simulink model "ofdm_13"  (Simulink 7.4)
settings: Solver=FixedStepDiscrete  SolverMode=SingleTasking  StartTime=0.0  StopTime=inf  MaxStep=1/(100*40e6)  RelTol=1e-3
PreLoadFcn:
  | Fsymbol              = .5e6;         % Symbol rate
  | D=8;  % decimation / interpolation
  | Bits_per_Symbol = 2;
  | Fbit  = Bits_per_Symbol*Fsymbol;
  | 
  | FFT_Size  = 64;
  | Cyclic        = 16;
  | Pilots         = 16;
  | Pilot_Level = 8;
  | Zero_Pad  = 3;
  | QAM_Level = 6;
  | 
  | OFDM_Frame =  FFT_Size+Cyclic;
  | Symbols_per_Frame = FFT_Size-Pilots-Zero_Pad;
  | 
  | Bits_per_Frame = Bits_per_Symbol*Symbols_per_Frame;
  | 
  | F_nco = Fsymbol*D*OFDM_Frame/(Symbols_per_Frame);
  | nco_nominal=2/D;
  | 
  | 
  | Fdelay = 8;  % rrc filter delay
  | Alpha = .25;  % excess BW
  | rrc_coef=rcosine(1,D,'fir/sqrt',Alpha,Fdelay);
  | rrc_coef=rrc_coef/sum(rrc_coef);
  | 
  | 
  | % coefficents for Farrow filter
  | b3 = [1/6 -1/2  1/2 -1/6];
  | b2 = [1/2 -1    1/2  0];
  | b1 = [1/3  1/2 -1    1/6];
  | b0 = [0    1    0    0];
StartFcn:
  | tic
StopFcn:
  | trun=toc
values from neighbouring files (symbols this model uses):
  Fs = 1    [16 qam.m]    (also in G.m = input('Enter sampling frequency='))
  j = imread('lena.jpg')    [ansk3.m]    (also in cosine_filter.m = 2; imag1.m)
  N = [N1;N2;N1_;N2_]    [FFT_OFDM_MIMO.m]    (also in MRCplot.m = 1000000; SDplot.m = 1000000; ansk2.m = 10; ansk3.m = 10)
undefined symbols (not defined in the file or in its folder): dBW, dfilt, Hz, magnitude, sided, Ts, Two
libraries: simulink x25, dspobslib x22, dspsigops x13, dspbuff3 x5, dspsnks4 x4, dspxfrm3 x4, dspstat3 x4, commsink2 x3, commchan3 x2, dsparch4 x2, commrandsrc2 x2, commdigbbndam3 x2
(part 1 of 2)
Description:
  | Pilot Driven OFDM  Synchronization
settings Model: Creator=Dick Benson  LastModifiedBy=Dick
settings Model: ModifiedHistory=|
  | 12/8/07  D&C
  | 12/03/08  Added BER, tuned control loops, enhanced channel model.
settings DataIOCC: SaveOutput=off  SignalLogging=off  SaveTime=off  SignalLoggingName=sigsOut
settings OptimizationCC: BlockReduction=off  BooleanDataType=off  InlineInvariantSignals=on  InitFltsAndDblsToZero=on
settings DebuggingCC: SaveWithParameterizedLinksMsg=none  SignalResolutionControl=TryResolveAllWithWarning  SolverPrmCheckMsg=none  InheritedTsInSrcMsg=none  MultiTaskDSMMsg=warning  MultiTaskCondExecSysMsg=none  ParameterPrecisionLossMsg=none  StrictBusMsg=None
settings HardwareCC: TargetUnknown=on
settings RTWCC: IncludeERTFirstTime=on
settings GRTTargetCC: TargetFcnLib=ansi_tfl_tmw.mat

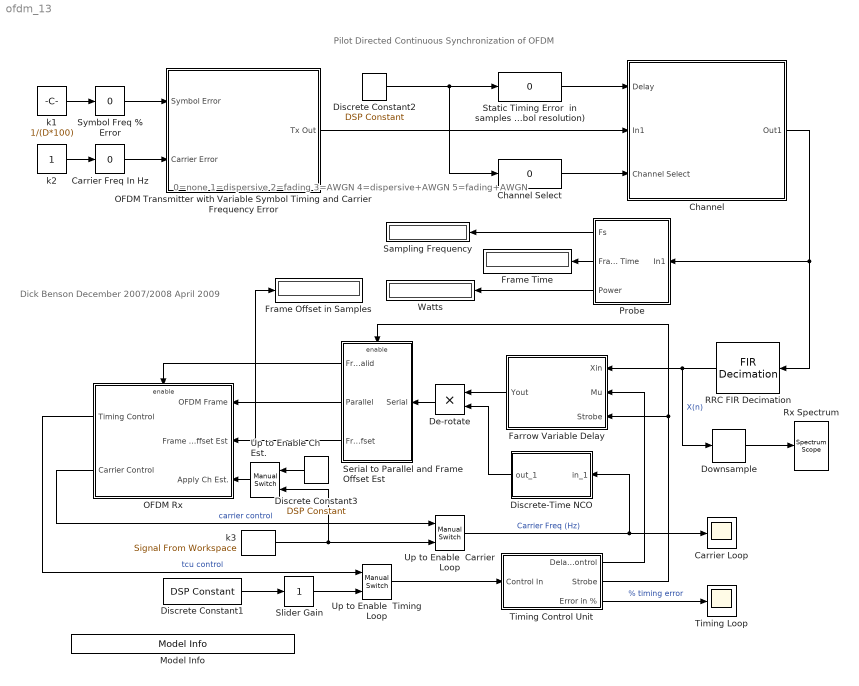
== system ofdm_13 ==
  note: Pilot Directed Continuous Synchronization of OFDM
  note: Dick Benson
      | December 2007/2008
      | April 2009
  note: 0=none
      | 1=dispersive
      | 2=fading
      | 3=AWGN
      | 4=dispersive+AWGN
      | 5=fading+AWGN
  Carrier Freq In Hz : simulink/Math Operations/Slider Gain  SystemSampleTime=-1  low=-1000  gain=0  high=1000
  Carrier Loop : Scope
      settings: TimeRange=0.008999999999999999  YMin=-1000  YMax=1000  MaxDataPoints=50000  Decimation=4
  Channel : Subsystem
  Channel Select : simulink/Math Operations/Slider Gain  SystemSampleTime=-1  low=0  gain=0  high=5
  De-rotate : Product  OutDataType=sfix(16)  OutScaling=2^0  RndMeth=Zero
  Discrete Constant1 : dspobslib/DSP Constant  SystemSampleTime=-1  Value=nco_nominal  SampleMode=Discrete  discreteOutput=Sample-based (interpret vectors as 1-D)  continuousOutput=Sample-based  sampTime=2/F_nco  framePeriod=2/F_nco  dataType=Inherit via back propagation  isSigned=on  wordLen=16  udDataType=sfix(16)  fracBitsMode=Best precision  numFracBits=15  InterpretAs1D=on  Ts=2/F_nco  FramebasedOutput=off
      settings: additionalParams=on
  Discrete Constant2 : dspobslib/DSP Constant  SystemSampleTime=-1  Value=1  SampleMode=Discrete  discreteOutput=Sample-based (interpret vectors as 1-D)  continuousOutput=Sample-based  sampTime=inf  framePeriod=inf  dataType=Inherit via back propagation  isSigned=on  wordLen=16  udDataType=sfix(16)  fracBitsMode=Best precision  numFracBits=15  InterpretAs1D=on  Ts=inf  FramebasedOutput=off
      settings: additionalParams=on
  Discrete Constant3 : dspobslib/DSP Constant  SystemSampleTime=-1  Value=1  SampleMode=Discrete  discreteOutput=Sample-based (interpret vectors as 1-D)  continuousOutput=Sample-based  sampTime=inf  framePeriod=inf  dataType=Inherit via back propagation  isSigned=on  wordLen=16  udDataType=sfix(16)  fracBitsMode=Best precision  numFracBits=15  InterpretAs1D=on  Ts=inf  FramebasedOutput=off
      settings: additionalParams=on
  Discrete-Time NCO : Subsystem  mask(Discrete-Time VCO){Ac=1, Fc=0, Kc=1, Ph=0, ts=2/F_nco}
      mask prompts: Ac "Output amplitude:"; Fc "Oscillation frequency (Hz):"; Kc "Input sensitivity:"; Ph "Initial phase (rad):"; ts "Sample time:"
      mask help: Generate a discrete-time output signal whose frequency changes in response to the amplitude variations of the input signal. The input signal must be a scalar.
      mask init:
      | if ((length(Ac)~=1) | (length(Fc)~=1) | (length(Kc)~=1) | (length(Ph)~=1) | (length(ts)~=1) |(length(Ph)~=1))error('Mask parameters must be scalar values.');end;
      | pi2=2*pi;
      mask Help: helpview(commbhelp)
      mask Display: disp('Discrete-Time\nNCO (rab)')
  Downsample : dspsigops/Downsample  N=D/2  phase=0  ic=0  smode=Allow multirate  fmode=Maintain input frame size
  Farrow Variable Delay : Subsystem
  Frame Offset in Samples : Display
  Frame Time : Display
  Model Info : simulink/Model-Wide Utilities/Model Info  SystemSampleTime=-1  InitialBlockCM=none  BlockCM=none  Frame=on  DisplayStringWithTags=Copywrite 2008-2010 The MathWorks, Inc.  HorizontalTextAlignment=Center  LeftAlignmentValue=0.5  SourceBlockDiagram=ofdm_13  TagMaxNumber=20
  OFDM Rx : Subsystem
  OFDM Transmitter with Variable Symbol Timing and Carrier Frequency Error : Subsystem
  Probe : Subsystem
  RRC FIR Decimation : dspmlti4/FIR Decimation  DialogController=dspdialog.FIRDecimation  DialogControllerArgs=DataTag16  h=rrc_coef  D=D/4  filtStruct=Direct form  framing=Maintain input frame rate  outputBufInitCond=0  roundingMode=Floor  overflowMode=off  FilterSource=Specify via dialog  FilterObject=Hm_firdecim
  Rx Spectrum : dspsnks4/Spectrum Scope  DialogController=dspdialog.SpectrumScope  DialogControllerArgs=DataTag17  SystemSampleTime=-1  ScopeProperties=on  Domain=Frequency  HorizSpan=1  UseBuffer=on  BufferSize=80  Overlap=0  inpFftLenInherit=on  FFTlength=256  numAvg=10  DisplayProperties=off  AxisGrid=on  Memory=off  FrameNumber=on  AxisLegend=off  AxisZoom=off  OpenScopeAtSimStart=on  OpenScopeImmediately=off  FigPos=[623 549 194 174]  AxisProperties=off  XUnits=Hertz  XRange=Two-sided ((-Fs/2...Fs/2])  XDisplay=0  InheritXIncr=on  XIncr=1.0  XLabel=Samples  XLimit=Auto  YUnits=dBW/Hertz  XMax=1  XMin=0  YLabel=dBW/Hz  LineProperties=off  wintypeSpecScope=Boxcar  RsSpecScope=50  betaSpecScope=5  winsampSpecScope=Periodic  XAxisParamsVer=6.8
      settings: YMin=-79.4885  YMax=-44.4885
  Sampling Frequency : Display
  Serial to Parallel and Frame Offset Est : Subsystem  TreatAsAtomicUnit=on
  Slider Gain : simulink/Math Operations/Slider Gain  SystemSampleTime=-1  low=0.99  gain=1  high=1.01
  Static Timing Error  in samples (1/8 symbol resolution) : simulink/Math Operations/Slider Gain  SystemSampleTime=-1  low=-40  gain=0  high=40
  "Symbol Freq % Error " : simulink/Math Operations/Slider Gain  SystemSampleTime=-1  low=-0.5  gain=0  high=0.5
  Timing Control Unit : Subsystem
  Timing Loop : Scope
      settings: TimeRange=0.008999999999999999  YMin=-0.5  YMax=0.5  MaxDataPoints=50000
  Up to Enable  Carrier Loop : simulink/Signal Routing/Manual Switch  SystemSampleTime=-1  sw=0  action=0  varsize=off
  Up to Enable Ch Est. : simulink/Signal Routing/Manual Switch  SystemSampleTime=-1  sw=0  action=0  varsize=off
  Up to Enable  Timing Loop : simulink/Signal Routing/Manual Switch  SystemSampleTime=-1  sw=0  action=0  varsize=off
  Watts : Display
  k1 : Constant  Value=1/(D*100)  OutDataType=sfix(16)  OutScaling=2^0
  k2 : Constant  OutDataType=sfix(16)  OutScaling=2^0
  k3 : dspsrcs4/Signal From Workspace  SystemSampleTime=-1  X=0  Ts=-1  nsamps=1  OutputAfterFinalValue=Holding final value  ignoreOrWarnInputAndFrameLengths=off
  wires:
  k1/1 -> "Symbol Freq % Error "/1
  "Symbol Freq % Error "/1 -> OFDM Transmitter with Variable Symbol Timing and Carrier Frequency Error/1(Symbol Error)
  Carrier Freq In Hz/1 -> OFDM Transmitter with Variable Symbol Timing and Carrier Frequency Error/2(Carrier Error)
  k2/1 -> Carrier Freq In Hz/1
  Probe/1(Fs) -> Sampling Frequency/1
  OFDM Transmitter with Variable Symbol Timing and Carrier Frequency Error/1(Tx Out) -> Channel/2(In1)
  Timing Control Unit/1(Delay Control) -> Farrow Variable Delay/2(Mu)
  Timing Control Unit/2(Strobe) -> Farrow Variable Delay/3(Strobe), Serial to Parallel and Frame Offset Est/Enable
  Discrete Constant1/1 -> Slider Gain/1
  RRC FIR Decimation/1 -> Farrow Variable Delay/1(Xin), Downsample/1  "X(n)"
  Channel/1(Out1) -> RRC FIR Decimation/1, Probe/1(In1)
  Probe/3(Power) -> Watts/1
  Probe/2(Frame Time) -> Frame Time/1
  Discrete Constant2/1 -> Static Timing Error  in samples (1/8 symbol resolution)/1, Channel Select/1
  Static Timing Error  in samples (1/8 symbol resolution)/1 -> Channel/1(Delay)
  OFDM Rx/1(Timing Control) -> Up to Enable  Timing Loop/1  "tcu control"
  Up to Enable  Timing Loop/1 -> Timing Control Unit/1(Control In)
  Discrete-Time NCO/1(out_1) -> De-rotate/2
  De-rotate/1 -> Serial to Parallel and Frame Offset Est/1(Serial)
  Farrow Variable Delay/1(Yout) -> De-rotate/1
  Timing Control Unit/3(Error in %) -> Timing Loop/1  "% timing error"
  Downsample/1 -> Rx Spectrum/1
  Serial to Parallel and Frame Offset Est/2(Parallel) -> OFDM Rx/1(OFDM Frame)
  Serial to Parallel and Frame Offset Est/3(Frame Offset) -> OFDM Rx/2(Frame Offset Est), Frame Offset in Samples/1
  Slider Gain/1 -> Up to Enable  Timing Loop/2
  OFDM Rx/2(Carrier Control) -> Up to Enable  Carrier Loop/1  "carrier control"
  Up to Enable  Carrier Loop/1 -> Discrete-Time NCO/1(in_1), Carrier Loop/1  "Carrier Freq (Hz)"
  k3/1 -> Up to Enable  Carrier Loop/2, Up to Enable Ch Est./2
  Serial to Parallel and Frame Offset Est/1(FrameValid) -> OFDM Rx/Enable
  Up to Enable Ch Est./1 -> OFDM Rx/3(Apply Ch Est.)
  Discrete Constant3/1 -> Up to Enable Ch Est./1
  Channel Select/1 -> Channel/3(Channel Select)

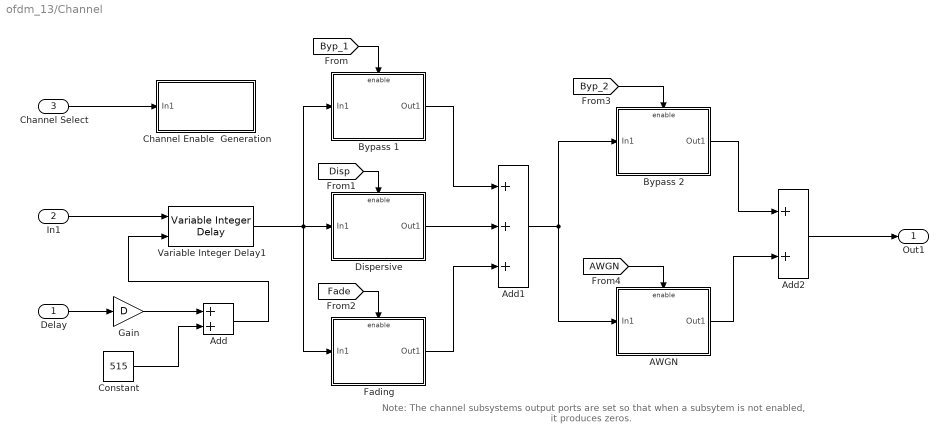
== system ofdm_13/Channel ==
  note: Note: The channel subsystems output ports are set so that
      | when a subsytem is not enabled, it produces zeros.
  Delay : Inport  OutDataType=sfix(16)  OutScaling=2^0
  In1 : Inport  Port=2  OutDataType=sfix(16)  OutScaling=2^0
  Channel Select : Inport  Port=3  OutDataType=sfix(16)  OutScaling=2^0
  AWGN : Subsystem  TreatAsAtomicUnit=on
  Add : Sum  OutDataType=sfix(16)  OutScaling=2^-10
  Add1 : Sum  Inputs=+++  OutDataType=sfix(16)  OutScaling=2^-10
  Add2 : Sum  OutDataType=sfix(16)  OutScaling=2^-10
  Bypass 1 : Subsystem  TreatAsAtomicUnit=on
  Bypass 2 : Subsystem  TreatAsAtomicUnit=on
  Channel Enable  Generation : Subsystem
  Constant : Constant  Value=515  OutDataType=sfix(16)  OutScaling=2^0
  Dispersive : Subsystem  TreatAsAtomicUnit=on
  Fading : Subsystem  TreatAsAtomicUnit=on
  Gain : Gain  Gain=D  ParameterDataType=sfix(16)  ParameterScaling=2^0  OutDataType=sfix(16)  OutScaling=2^0
  Variable Integer Delay1 : dspsigops/Variable Integer Delay  dmax=2*516  ic=0  noDFT=off
  Out1 : Outport  OutDataType=sfix(16)  OutScaling=2^0
  wires:
  Delay/1 -> Gain/1
  Constant/1 -> Add/2
  Gain/1 -> Add/1
  Dispersive/1(Out1) -> Add1/2
  Bypass 1/1(Out1) -> Add1/1
  Fading/1(Out1) -> Add1/3
  Add1/1 -> AWGN/1(In1), Bypass 2/1(In1)
  Bypass 2/1(Out1) -> Add2/1
  AWGN/1(Out1) -> Add2/2
  Add2/1 -> Out1/1
  Channel Select/1 -> Channel Enable  Generation/1(In1)
  [Byp_1] -> Bypass 1/Enable
  [Disp] -> Dispersive/Enable
  [Fade] -> Fading/Enable
  [Byp_2] -> Bypass 2/Enable
  [AWGN] -> AWGN/Enable
  Variable Integer Delay1/1 -> Dispersive/1(In1), Bypass 1/1(In1), Fading/1(In1)
  In1/1 -> Variable Integer Delay1/1
  Add/1 -> Variable Integer Delay1/2

== system ofdm_13/Discrete-Time NCO ==
  note: Amplitude
  note: Phase Accumulator
      | Modulus
  note: Center Freq
  note: VCO Sensitivity
  note: initial condx=Ph
  in_1 : Inport  OutDataType=sfix(16)  OutScaling=2^0
  Discrete Constant1 : dspobslib/DSP Constant  SystemSampleTime=-1  Value=Fc*pi2*ts  SampleMode=Discrete  discreteOutput=Sample-based (interpret vectors as 1-D)  continuousOutput=Sample-based  sampTime=ts  framePeriod=ts  dataType=Inherit via back propagation  isSigned=on  wordLen=16  udDataType=sfix(16)  fracBitsMode=Best precision  numFracBits=15  InterpretAs1D=on  Ts=ts  FramebasedOutput=off
      settings: additionalParams=on
  Discrete Constant2 : dspobslib/DSP Constant  SystemSampleTime=-1  Value=pi2  SampleMode=Discrete  discreteOutput=Sample-based (interpret vectors as 1-D)  continuousOutput=Sample-based  sampTime=ts  framePeriod=ts  dataType=Inherit via back propagation  isSigned=on  wordLen=16  udDataType=sfix(16)  fracBitsMode=Best precision  numFracBits=15  InterpretAs1D=on  Ts=ts  FramebasedOutput=off
      settings: additionalParams=on
  Math Function : Math  Operator=mod  OutDataType=sfix(16)  OutScaling=2^0  SaturateOnIntegerOverflow=on
  Real-Imag to Complex : RealImagToComplex
  Sensitivity : Gain  Gain=Kc*pi2*ts  ParameterDataType=sfix(16)  ParameterScaling=2^0  OutDataType=sfix(16)  OutScaling=2^0  SaturateOnIntegerOverflow=on  OutDataTypeStr=Inherit: Same as input  ParamDataTypeStr=Inherit: Same as input
  Sensitivity2 : Gain  Gain=Ac  ParameterDataType=sfix(16)  ParameterScaling=2^0  OutDataType=sfix(16)  OutScaling=2^0  SaturateOnIntegerOverflow=on  OutDataTypeStr=Inherit: Same as input  ParamDataTypeStr=Inherit: Same as input
  Sum1 : Sum  Inputs=+++  OutDataType=sfix(16)  OutScaling=2^0  SaturateOnIntegerOverflow=on  InputSameDT=on  OutDataTypeStr=Inherit: Same as first input
  Trigonometric Function : Trigonometry  Operator=cos
  Trigonometric Function1 : Trigonometry
  Unit Delay : UnitDelay  X0=Ph  SampleTime=ts
  out_1 : Outport  OutDataType=sfix(16)  OutScaling=2^0  InitialOutput=0
  wires:
  Discrete Constant1/1 -> Sum1/2
  Sensitivity2/1 -> out_1/1
  Trigonometric Function/1 -> Real-Imag to Complex/1
  Unit Delay/1 -> Sum1/3, Trigonometric Function1/1, Trigonometric Function/1
  Sensitivity/1 -> Sum1/1
  in_1/1 -> Sensitivity/1
  Math Function/1 -> Unit Delay/1
  Sum1/1 -> Math Function/1
  Discrete Constant2/1 -> Math Function/2
  Trigonometric Function1/1 -> Real-Imag to Complex/2
  Real-Imag to Complex/1 -> Sensitivity2/1

== system ofdm_13/Farrow Variable Delay ==
  Xin : Inport  OutDataType=sfix(16)  OutScaling=2^0
  Mu : Inport  Port=2  OutDataType=sfix(16)  OutScaling=2^0
  Strobe : Inport  Port=3  OutDataType=sfix(16)  OutScaling=2^0
  Calculate Filter : Subsystem
  Filter State (4x1) : dspbuff3/Buffer  N=4  V=3  ic=0
  Yout : Outport  OutDataType=sfix(16)  OutScaling=2^0
  wires:
  Xin/1 -> Filter State (4x1)/1
  Mu/1 -> Calculate Filter/1(In1)
  Filter State (4x1)/1 -> Calculate Filter/2(In2)
  Calculate Filter/1(Out1) -> Yout/1
  Strobe/1 -> Calculate Filter/Enable

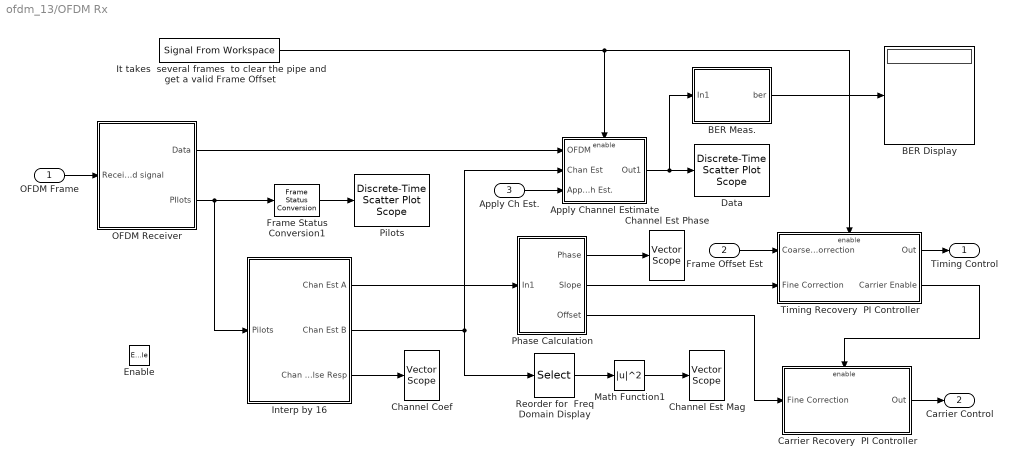
== system ofdm_13/OFDM Rx ==
  OFDM Frame : Inport  OutDataType=sfix(16)  OutScaling=2^0
  Frame Offset Est : Inport  Port=2  OutDataType=sfix(16)  OutScaling=2^0
  Apply Ch Est. : Inport  Port=3  OutDataType=sfix(16)  OutScaling=2^0
  Enable : EnablePort
  Apply Channel Estimate : Subsystem
  BER Display : Display
  BER Meas. : Subsystem
  Carrier Recovery  PI Controller : Subsystem
  Channel Coef : dspsnks4/Vector Scope  DialogController=dspdialog.VectorScope  DialogControllerArgs=DataTag3  ScopeProperties=on  Domain=Time  HorizSpan=1  DisplayProperties=off  AxisGrid=on  Memory=off  FrameNumber=off  AxisLegend=off  AxisZoom=off  OpenScopeAtSimStart=on  OpenScopeImmediately=off  FigPos=[827 549 193 173]  AxisProperties=off  XUnits=Hertz  XRange=[0...Fs/2]  InheritXIncr=on  XIncr=1  XLabel=Time  XLimit=Auto  XMin=0  XMax=1  XStart=0  YUnits=dB  YLabel=Amplitude  LineProperties=off  LineStyles=none|none  LineMarkers=*|*  LineColors=blue | red  XAxisParamsVer=6.8
      settings: YMin=-2  YMax=2
  "Channel Est Mag " : dspsnks4/Vector Scope  DialogController=dspdialog.VectorScope  DialogControllerArgs=DataTag4  ScopeProperties=on  Domain=Frequency  HorizSpan=1  DisplayProperties=off  AxisGrid=on  Memory=off  FrameNumber=on  AxisLegend=off  AxisZoom=off  OpenScopeAtSimStart=on  OpenScopeImmediately=off  FigPos=[624 329 193 172]  AxisProperties=off  XUnits=Hertz  XRange=[-Fs/2...Fs/2]  InheritXIncr=off  XIncr=8/F_nco  XLabel=Time  XLimit=Auto  XMin=0  XMax=1  XStart=0  YUnits=dB  YLabel=Amplitude in dB  LineProperties=off  XAxisParamsVer=6.8
      settings: YMin=-20  YMax=15
  Channel Est Phase : dspsnks4/Vector Scope  DialogController=dspdialog.VectorScope  DialogControllerArgs=DataTag5  ScopeProperties=on  Domain=Frequency  HorizSpan=1  DisplayProperties=off  AxisGrid=on  Memory=off  FrameNumber=off  AxisLegend=off  AxisZoom=off  OpenScopeAtSimStart=on  OpenScopeImmediately=off  FigPos=[827 332 196 169]  AxisProperties=off  XUnits=Hertz  XRange=[-Fs/2...Fs/2]  InheritXIncr=off  XIncr=8/F_nco  XLabel=Time  XLimit=Auto  XMin=0  XMax=1  XStart=0  YUnits=Magnitude  YLabel=Degrees  LineProperties=off  LineColors=blue  XAxisParamsVer=6.8
      settings: YMin=-400  YMax=400
  Data : commsink2/Discrete-Time Scatter Plot Scope  Tag=ScatterPlot  SystemSampleTime=-1  sampPerSymb=1  offsetEye=0  numTraces=100  numNewFrames=10  LineMarkers=square  LineColors=r  fading=off  render=off  AxisGrid=on  xMin=-2  xMax=2  yMin=-2  yMax=2  inphaseLabel=In-phase Amplitude  quadratureLabel=Quadrature Amplitude  openScopeAtSimStart=on  FrameNumber=off  FigPos=[626 82 194 198]  figTitle=Scatter Plot  numLinesMax=8  block_type_=scatter
  Frame Status Conversion1 : dspobslib/Frame Status Conversion  SystemSampleTime=-1  growRefPort=off  outframe=Frame-based
  Interp by 16 : Subsystem
  It takes  several frames  to clear the pipe and get a valid Frame Offset : dspsrcs4/Signal From Workspace  SystemSampleTime=-1  X=[zeros(1,10),1]  Ts=-1  nsamps=1  OutputAfterFinalValue=Holding final value  ignoreOrWarnInputAndFrameLengths=off
  Math Function1 : Math  Operator=magnitude^2  OutDataType=sfix(16)  OutScaling=2^0  SaturateOnIntegerOverflow=on
  OFDM Receiver : Subsystem
      mask Display:
      | disp('OFDM\nReceiver');
      | port_label('output',2,'pilots')
  Phase Calculation : Subsystem
  Pilots : commsink2/Discrete-Time Scatter Plot Scope  Tag=ScatterPlot  SystemSampleTime=-1  sampPerSymb=1  offsetEye=0  numTraces=100  numNewFrames=10  LineMarkers=*  LineColors=r  fading=off  render=off  AxisGrid=on  xMin=-2  xMax=2  yMin=-2  yMax=2  inphaseLabel=In-phase Amplitude  quadratureLabel=Quadrature Amplitude  openScopeAtSimStart=on  FrameNumber=off  FigPos=[828 84 191 197]  figTitle=Scatter Plot  numLinesMax=8  block_type_=scatter
  Reorder for  Freq Domain Display : Selector  InputPortWidth=64  IndexOptions=Index vector (dialog)  Indices=[33:64 1:32]  OutputSizes=1
  Timing Recovery  PI Controller : Subsystem
  Timing Control : Outport  OutDataType=sfix(16)  OutScaling=2^0  InitialOutput=nco_nominal
  Carrier Control : Outport  Port=2  OutDataType=sfix(16)  OutScaling=2^0  InitialOutput=0
  wires:
  OFDM Frame/1 -> OFDM Receiver/1(Received signal)
  OFDM Receiver/2(PIlots) -> Interp by 16/1(Pilots), Frame Status Conversion1/1
  Interp by 16/2(Chan Est B) -> Apply Channel Estimate/2(Chan Est), Reorder for  Freq Domain Display/1
  Reorder for  Freq Domain Display/1 -> Math Function1/1
  Phase Calculation/2(Slope) -> Timing Recovery  PI Controller/2(Fine Correction)
  OFDM Receiver/1(Data) -> Apply Channel Estimate/1(OFDM)
  Phase Calculation/1(Phase) -> Channel Est Phase/1
  Math Function1/1 -> "Channel Est Mag "/1
  Timing Recovery  PI Controller/1(Out) -> Timing Control/1
  It takes  several frames  to clear the pipe and get a valid Frame Offset/1 -> Apply Channel Estimate/Enable, Timing Recovery  PI Controller/Enable
  Carrier Recovery  PI Controller/1(Out) -> Carrier Control/1
  Frame Offset Est/1 -> Timing Recovery  PI Controller/1(Coarse Correction)
  Phase Calculation/3(Offset) -> Carrier Recovery  PI Controller/1(Fine Correction)
  Interp by 16/3(Chan Impulse Resp) -> Channel Coef/1
  Interp by 16/1(Chan Est A) -> Phase Calculation/1(In1)
  Frame Status Conversion1/1 -> Pilots/1
  Apply Channel Estimate/1(Out1) -> Data/1, BER Meas./1(In1)
  Apply Ch Est./1 -> Apply Channel Estimate/3(Apply Ch Est.)
  Timing Recovery  PI Controller/2(Carrier Enable) -> Carrier Recovery  PI Controller/Enable
  BER Meas./1(ber) -> BER Display/1

== system ofdm_13/OFDM Transmitter with Variable Symbol Timing and Carrier Frequency Error ==
  note: Use Farrow Fractional Delay and NCO to create Tx with variable symbol rate.
  Symbol Error : Inport  OutDataType=sfix(16)  OutScaling=2^0
  Carrier Error : Inport  Port=2  OutDataType=sfix(16)  OutScaling=2^0
  Buffer : dspbuff3/Buffer  N=OFDM_Frame*D  V=0  ic=0
  Buffer1 : dspbuff3/Buffer  N=OFDM_Frame*D  V=0  ic=0
  "Digital Filter RRC " : dsparch4/Digital Filter  DialogController=dspdialog.DigitalFilter  DialogControllerArgs=DataTag11  TypePopup=FIR (all zeros)  IIRFiltStruct=Direct form II transposed  AllPoleFiltStruct=Direct form  FIRFiltStruct=Direct form  CoeffSource=Specify via dialog  NumCoeffs=rrc_coef  DenCoeffs=[1 0.1]  BiQuadCoeffs=[1 0.3 0.4 1 0.1 0.2]  LatticeCoeffs=[0.2 0.4]  denIgnore=on  FiltPerSampPopup=One filter per frame  IC=0  ICnum=0  ICden=0  roundingMode=Floor  overflowMode=off  ScaleValues=1  scaleValueFracLength=14  stageInFracLength=15  stageOutFracLength=15  FilterSource=Specify via dialog  dfiltObjectName=dfilt.dffir([1 2 1])
  Discrete Constant1 : dspobslib/DSP Constant  SystemSampleTime=-1  Value=1/D  SampleMode=Discrete  discreteOutput=Sample-based (interpret vectors as 1-D)  continuousOutput=Sample-based  sampTime=inf  framePeriod=inf  dataType=Inherit via back propagation  isSigned=on  wordLen=16  udDataType=sfix(16)  fracBitsMode=Best precision  numFracBits=15  InterpretAs1D=on  Ts=inf  FramebasedOutput=off
      settings: additionalParams=on
  Discrete-Time NCO : Subsystem  mask(Discrete-Time VCO){Ac=1, Fc=0, Kc=1, Ph=0, ts=1/F_nco}
      mask prompts: Ac "Output amplitude:"; Fc "Oscillation frequency (Hz):"; Kc "Input sensitivity:"; Ph "Initial phase (rad):"; ts "Sample time:"
      mask help: Generate a discrete-time output signal whose frequency changes in response to the amplitude variations of the input signal. The input signal must be a scalar.
      mask init:
      | if ((length(Ac)~=1) | (length(Fc)~=1) | (length(Kc)~=1) | (length(Ph)~=1) | (length(ts)~=1) |(length(Ph)~=1))error('Mask parameters must be scalar values.');end;
      | pi2=2*pi;
      mask Help: helpview(commbhelp)
      mask Display: disp('Discrete-Time\nNCO (rab)')
  Farrow Variable Delay : Subsystem
  OFDM Symbol Gen : Subsystem
  Rotate : Product  OutDataType=sfix(16)  OutScaling=2^0  RndMeth=Zero
  Sum2 : Sum  OutDataType=sfix(16)  OutScaling=2^0  SaturateOnIntegerOverflow=on  InputSameDT=on  OutDataTypeStr=Inherit: Same as first input
  Timing Control Unit1 : Subsystem
  Tx Out : Outport  OutDataType=sfix(16)  OutScaling=2^0
  wires:
  Rotate/1 -> Tx Out/1
  Symbol Error/1 -> Sum2/1
  Farrow Variable Delay/1(Yout) -> Buffer/1
  Buffer/1 -> "Digital Filter RRC "/1
  "Digital Filter RRC "/1 -> Rotate/1
  Discrete-Time NCO/1(out_1) -> Buffer1/1
  Carrier Error/1 -> Discrete-Time NCO/1(in_1)
  Buffer1/1 -> Rotate/2
  Sum2/1 -> Timing Control Unit1/1(Control In)
  Timing Control Unit1/2(Delay Control) -> Farrow Variable Delay/2(Mu)
  Timing Control Unit1/1(Clock Out) -> OFDM Symbol Gen/Enable
  Discrete Constant1/1 -> Sum2/2
  OFDM Symbol Gen/1(Serial Samples Out) -> Farrow Variable Delay/1(Xin)

== system ofdm_13/Probe ==
  In1 : Inport  OutDataType=sfix(16)  OutScaling=2^0
  Divide : Product  Inputs=/*  OutDataType=sfix(16)  OutScaling=2^-10
  Probe : Probe  ProbeWidth=off  ProbeComplexSignal=off  ProbeSignalDimensions=on
  Selector : Selector  InputPortWidth=2  IndexOptions=Index vector (dialog)  Indices=[1]  OutputSizes=1
  Selector1 : Selector  InputPortWidth=2  IndexOptions=Index vector (dialog)  Indices=[1]  OutputSizes=1
  Variance : dspstat3/Variance  DialogController=dspDDGCreate  DialogControllerArgs=DataTag15  run=off  reset_popup=None  directionMode=Each column  dimension=1  treatSBRowAsCol=on  roiEnable=off  roiType=Rectangles  roiPortion=Entire ROI  roiOutput=Individual statistics for each ROI  roiFlag=off  roundingMode=Floor  overflowMode=off
  Fs : Outport  OutDataType=sfix(16)  OutScaling=2^0
  Frame Time : Outport  Port=2  OutDataType=sfix(16)  OutScaling=2^0
  Power : Outport  Port=3  OutDataType=sfix(16)  OutScaling=2^0
  wires:
  In1/1 -> Probe/1, Variance/1
  Divide/1 -> Fs/1
  Selector/1 -> Divide/2
  Selector1/1 -> Divide/1, Frame Time/1
  Probe/1 -> Selector1/1
  Probe/2 -> Selector/1
  Variance/1 -> Power/1

== system ofdm_13/Serial to Parallel and Frame Offset Est ==
  note: This output is only
      | useful during the "FrameValid" signal.
  Serial : Inport  OutDataType=sfix(16)  OutScaling=2^0
  Enable : EnablePort
  Compare To Constant : simulink/Logic and Bit Operations/Compare To Constant  SystemSampleTime=-1  relop===  const=(OFDM_Frame-1)  LogicOutDataTypeMode=boolean  ZeroCross=off
  Counter Limited : simulink/Sources/Counter Limited  SystemSampleTime=-1  uplimit=(OFDM_Frame-1)  tsamp=-1
  Cyclic Prefix Correlation for Frame  Boundary Estimation : Subsystem
  Delay Line : dspbuff3/Delay Line  siz=OFDM_Frame  ic=0  directfeed=on  enable_output=off  hold_output=off
  FrameValid : Outport  OutDataType=sfix(16)  OutScaling=2^0  OutputWhenDisabled=reset  InitialOutput=0
  Parallel : Outport  Port=2  OutDataType=sfix(16)  OutScaling=2^0
  Frame Offset : Outport  Port=3  OutDataType=sfix(16)  OutScaling=2^0
  wires:
  Serial/1 -> Delay Line/1, Cyclic Prefix Correlation for Frame  Boundary Estimation/2(Serial)
  Counter Limited/1 -> Compare To Constant/1
  Delay Line/1 -> Parallel/1
  Compare To Constant/1 -> FrameValid/1, Cyclic Prefix Correlation for Frame  Boundary Estimation/1(Strobe)
  Cyclic Prefix Correlation for Frame  Boundary Estimation/1(Offset in Samples) -> Frame Offset/1

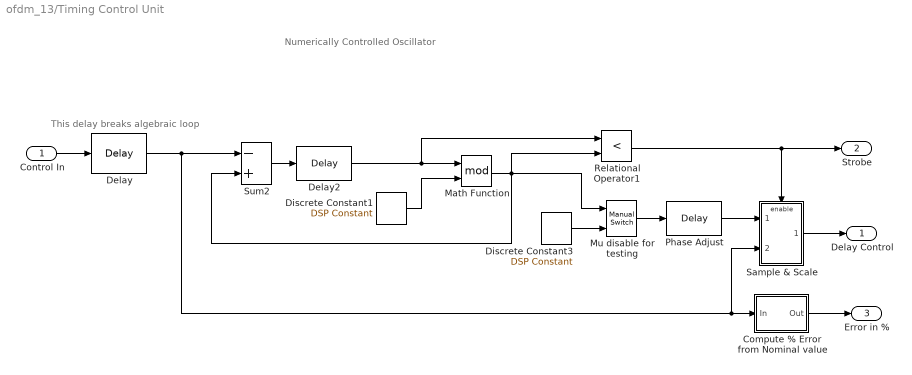
== system ofdm_13/Timing Control Unit ==
  note: Numerically Controlled Oscillator
  note: This delay breaks algebraic loop
  Control In : Inport  OutDataType=sfix(16)  OutScaling=2^0
  Compute % Error from Nominal value : Subsystem
  Delay : dspsigops/Delay  dly_unit=Samples  delay=1  ic_detail=off  dif_ic_for_ch=off  dif_ic_for_dly=off  ic=nco_nominal  reset_popup=None
  Delay2 : dspsigops/Delay  dly_unit=Samples  delay=1  ic_detail=on  dif_ic_for_ch=off  dif_ic_for_dly=off  ic=0  reset_popup=None
  Discrete Constant1 : dspobslib/DSP Constant  SystemSampleTime=-1  Value=1  SampleMode=Discrete  discreteOutput=Sample-based (interpret vectors as 1-D)  continuousOutput=Sample-based  sampTime=inf  framePeriod=inf  dataType=Inherit via back propagation  isSigned=on  wordLen=16  udDataType=sfix(16)  fracBitsMode=Best precision  numFracBits=15  InterpretAs1D=on  Ts=inf  FramebasedOutput=off
      settings: additionalParams=on
  Discrete Constant3 : dspobslib/DSP Constant  SystemSampleTime=-1  Value=0  SampleMode=Discrete  discreteOutput=Sample-based (interpret vectors as 1-D)  continuousOutput=Sample-based  sampTime=inf  framePeriod=inf  dataType=Inherit via back propagation  isSigned=on  wordLen=16  udDataType=sfix(16)  fracBitsMode=Best precision  numFracBits=15  InterpretAs1D=on  Ts=inf  FramebasedOutput=off
      settings: additionalParams=on
  Math Function : Math  Operator=mod  OutDataType=sfix(16)  OutScaling=2^0  SaturateOnIntegerOverflow=on
  Mu disable for testing : simulink/Signal Routing/Manual Switch  SystemSampleTime=-1  sw=1  action=0  varsize=off
  Phase Adjust : dspsigops/Delay  dly_unit=Samples  delay=1  ic_detail=on  dif_ic_for_ch=off  dif_ic_for_dly=off  ic=0  reset_popup=None
  Relational Operator1 : RelationalOperator  Operator=<  LogicOutDataTypeMode=boolean  LogicDataType=double(64)  OutDataTypeStr=boolean
  Sample & Scale : Subsystem
  Sum2 : Sum  Inputs=-+  OutDataType=sfix(16)  OutScaling=2^0  SaturateOnIntegerOverflow=on  InputSameDT=on  OutDataTypeStr=Inherit: Same as first input
  Delay Control : Outport  OutDataType=sfix(16)  OutScaling=2^0
  Strobe : Outport  Port=2  OutDataType=sfix(16)  OutScaling=2^0
  Error in % : Outport  Port=3  OutDataType=sfix(16)  OutScaling=2^0
  wires:
  Relational Operator1/1 -> Sample & Scale/Enable, Strobe/1
  Math Function/1 -> Relational Operator1/2, Sum2/2, Mu disable for testing/1
  Sum2/1 -> Delay2/1
  Discrete Constant1/1 -> Math Function/2
  Delay2/1 -> Relational Operator1/1, Math Function/1
  Control In/1 -> Delay/1
  Mu disable for testing/1 -> Phase Adjust/1
  Sample & Scale/1(Out1) -> Delay Control/1
  Phase Adjust/1 -> Sample & Scale/1(In1)
  Discrete Constant3/1 -> Mu disable for testing/2
  Delay/1 -> Sum2/1, Sample & Scale/2(In2), Compute % Error from Nominal value/1(In)
  Compute % Error from Nominal value/1(Out) -> Error in %/1

== system ofdm_13/Channel/AWGN ==
  In1 : Inport  OutDataType=sfix(16)  OutScaling=2^0
  Enable : EnablePort
  AWGN Channel1 : commchan3/AWGN Channel  SystemSampleTime=-1  seed=15  noiseMode="Signal to noise ratio  (SNR)"  EbNodB=10  EsNodB=10  SNRdB=15  bitsPerSym=1  Ps=1  Tsym=1  variance=1
  Out1 : Outport  OutDataType=sfix(16)  OutScaling=2^0  OutputWhenDisabled=reset  InitialOutput=0+j*eps
  wires:
  In1/1 -> AWGN Channel1/1
  AWGN Channel1/1 -> Out1/1

== system ofdm_13/Channel/Bypass 1 ==
  In1 : Inport  OutDataType=sfix(16)  OutScaling=2^0
  Enable : EnablePort
  Out1 : Outport  OutDataType=sfix(16)  OutScaling=2^0  OutputWhenDisabled=reset  InitialOutput=0+j*eps
  wires:
  In1/1 -> Out1/1

== system ofdm_13/Channel/Bypass 2 ==
  In1 : Inport  OutDataType=sfix(16)  OutScaling=2^0
  Enable : EnablePort
  Out1 : Outport  OutDataType=sfix(16)  OutScaling=2^0  OutputWhenDisabled=reset  InitialOutput=0+j*eps
  wires:
  In1/1 -> Out1/1

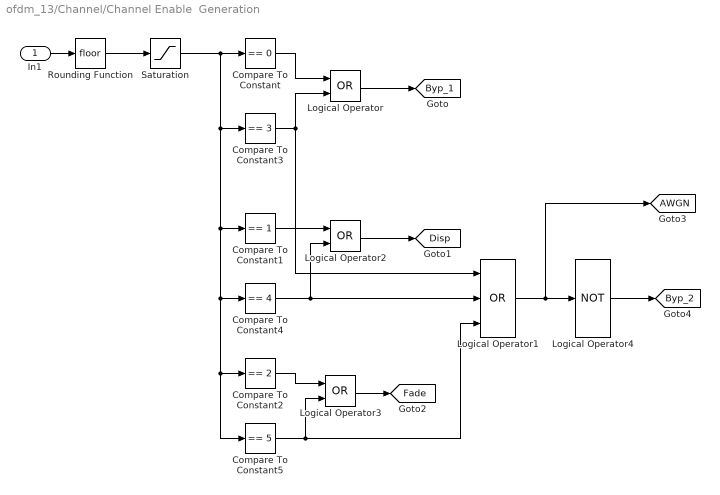
== system ofdm_13/Channel/Channel Enable  Generation ==
  In1 : Inport  OutDataType=sfix(16)  OutScaling=2^0
  Compare To Constant : simulink/Logic and Bit Operations/Compare To Constant  SystemSampleTime=-1  relop===  const=0  LogicOutDataTypeMode=boolean  ZeroCross=off
  Compare To Constant1 : simulink/Logic and Bit Operations/Compare To Constant  SystemSampleTime=-1  relop===  const=1  LogicOutDataTypeMode=boolean  ZeroCross=off
  Compare To Constant2 : simulink/Logic and Bit Operations/Compare To Constant  SystemSampleTime=-1  relop===  const=2  LogicOutDataTypeMode=boolean  ZeroCross=off
  Compare To Constant3 : simulink/Logic and Bit Operations/Compare To Constant  SystemSampleTime=-1  relop===  const=3  LogicOutDataTypeMode=boolean  ZeroCross=off
  Compare To Constant4 : simulink/Logic and Bit Operations/Compare To Constant  SystemSampleTime=-1  relop===  const=4  LogicOutDataTypeMode=boolean  ZeroCross=off
  Compare To Constant5 : simulink/Logic and Bit Operations/Compare To Constant  SystemSampleTime=-1  relop===  const=5  LogicOutDataTypeMode=boolean  ZeroCross=off
  Logical Operator : Logic  Operator=OR  AllPortsSameDT=off  OutDataTypeMode=boolean  OutDataTypeStr=boolean
  Logical Operator1 : Logic  Operator=OR  Inputs=3  AllPortsSameDT=off  OutDataTypeMode=boolean  OutDataTypeStr=boolean
  Logical Operator2 : Logic  Operator=OR  AllPortsSameDT=off  OutDataTypeMode=boolean  OutDataTypeStr=boolean
  Logical Operator3 : Logic  Operator=OR  AllPortsSameDT=off  OutDataTypeMode=boolean  OutDataTypeStr=boolean
  Logical Operator4 : Logic  Operator=NOT  Inputs=3  AllPortsSameDT=off  OutDataTypeMode=boolean  OutDataTypeStr=boolean
  Rounding Function : Rounding
  Saturation : Saturate  UpperLimit=5  LowerLimit=0  LinearizeAsGain=off  OutDataType=sfix(16)  OutScaling=2^0
  tag scope: AWGN=global, Byp_1=global, Byp_2=global, Disp=global, Fade=global
  wires:
  In1/1 -> Rounding Function/1
  Compare To Constant/1 -> Logical Operator/1
  Compare To Constant3/1 -> Logical Operator/2, Logical Operator1/1
  Logical Operator/1 -> [Byp_1]
  Compare To Constant4/1 -> Logical Operator1/2, Logical Operator2/2
  Compare To Constant5/1 -> Logical Operator1/3, Logical Operator3/2
  Compare To Constant1/1 -> Logical Operator2/1
  Logical Operator2/1 -> [Disp]
  Compare To Constant2/1 -> Logical Operator3/1
  Logical Operator3/1 -> [Fade]
  Logical Operator1/1 -> Logical Operator4/1, [AWGN]
  Logical Operator4/1 -> [Byp_2]
  Rounding Function/1 -> Saturation/1
  Saturation/1 -> Compare To Constant/1, Compare To Constant1/1, Compare To Constant4/1, Compare To Constant2/1, Compare To Constant5/1, Compare To Constant3/1

== system ofdm_13/Channel/Dispersive ==
  In1 : Inport  OutDataType=sfix(16)  OutScaling=2^0
  Enable : EnablePort
  Dispersive Channel : dsparch4/Digital Filter  DialogController=dspdialog.DigitalFilter  DialogControllerArgs=DataTag0  TypePopup=FIR (all zeros)  IIRFiltStruct=Direct form II transposed  AllPoleFiltStruct=Direct form  FIRFiltStruct=Direct form  CoeffSource=Specify via dialog  NumCoeffs="[1   0  0  0.8 0 0 0 -0.7      j*.500   0 0 0 0 0 0 0  -.5  0 0 0 0 0 0 0 0 .5]/1.8"  DenCoeffs=[1 0.1]  BiQuadCoeffs=[1 0.3 0.4 1 0.1 0.2]  LatticeCoeffs=[0.2 0.4]  denIgnore=on  FiltPerSampPopup=One filter per frame  IC=0  ICnum=0  ICden=0  roundingMode=Floor  overflowMode=off  ScaleValues=1  scaleValueFracLength=14  stageInFracLength=15  stageOutFracLength=15  FilterSource=Specify via dialog  dfiltObjectName=dfilt.dffir([1 2 1])
  Out1 : Outport  OutDataType=sfix(16)  OutScaling=2^0  OutputWhenDisabled=reset  InitialOutput=0+j*eps
  wires:
  Dispersive Channel/1 -> Out1/1
  In1/1 -> Dispersive Channel/1

== system ofdm_13/Channel/Fading ==
  In1 : Inport  OutDataType=sfix(16)  OutScaling=2^0
  Enable : EnablePort
  Multipath Rayleigh Fading Channel : commchan3/Multipath Rayleigh Fading Channel  SystemSampleTime=-1  maxDopplerShift=100  spectrumType=Jakes  sigmaGaussian=1/sqrt(2)  coeffRounded=[1 -1.72 0.785]  freqMinMaxRJakes=[0 1]  freqMinMaxAJakes=[0 1]  sigmaGaussian1=1/sqrt(2)  sigmaGaussian2=1/sqrt(2)  centerFreqGaussian1=0.0  centerFreqGaussian2=0.0  gainGaussian1=0.5  gainGaussian2=0.5  coeffBell=9  dopplerSpectrum=doppler.jakes  pathDelays=[0 1e-6, 3e-6]  avgPathGaindB=[0 -3, -6]  normalizePathGains=on  seed=73  enableProbe=0  openVisAtStart=off  outPathGains=off  outDelay=off
  Out1 : Outport  OutDataType=sfix(16)  OutScaling=2^0  OutputWhenDisabled=reset  InitialOutput=0+j*eps
  wires:
  In1/1 -> Multipath Rayleigh Fading Channel/1
  Multipath Rayleigh Fading Channel/1 -> Out1/1

== system ofdm_13/Farrow Variable Delay/Calculate Filter ==
  note: Filter Coefficients from Chris Dick Xilinx,
      | or H. Meyer pp 520 (9-33) Digital Communications Receivers
  In1 : Inport
  In2 : Inport  Port=2
  Enable : EnablePort
  Filter coefficients : Gain  Gain=fliplr([b3;b2;b1;b0])  Multiplication=Matrix(K*u)  ParameterDataType=sfix(16)  ParameterScaling=2^0  OutDataType=sfix(16)  OutScaling=2^0  SaturateOnIntegerOverflow=on  OutDataTypeStr=Inherit: Same as input  ParamDataTypeStr=Inherit: Same as input
  Polynomial Evaluation : dsppolyfun/Polynomial Evaluation  useConstCoeffs=off  constCoeffs=[5 4 3 2 1]
  Out1 : Outport
  wires:
  In1/1 -> Polynomial Evaluation/1
  Polynomial Evaluation/1 -> Out1/1
  In2/1 -> Filter coefficients/1
  Filter coefficients/1 -> Polynomial Evaluation/2

== system ofdm_13/OFDM Rx/Apply Channel Estimate ==
  note: Extract Matching Channel
      | Corrections
  OFDM : Inport
  Chan Est : Inport  Port=2
  Apply Ch Est. : Inport  Port=3  OutDataType=sfix(16)  OutScaling=2^0
  Enable : EnablePort
  Divide : Product  Inputs=*/  OutDataType=sfix(16)  OutScaling=2^0  RndMeth=Zero
  Frame Status Conversion2 : dspobslib/Frame Status Conversion  SystemSampleTime=-1  growRefPort=off  outframe=Frame-based
  Selector : Selector  InputPortWidth=64  IndexOptions=Index vector (dialog)  Indices="[  4:6   8:10  12:14  16:18  20:22  24:26  28:30   32:34  36:38    40:42     44:46   48:50  52:54  56:58   60:62   ]"  OutputSizes=1
  Switch : Switch  Threshold=.5  OutDataType=sfix(16)  OutScaling=2^0
  Out1 : Outport
  wires:
  Selector/1 -> Divide/2
  OFDM/1 -> Divide/1, Switch/3
  Chan Est/1 -> Selector/1
  Switch/1 -> Frame Status Conversion2/1
  Divide/1 -> Switch/1
  Apply Ch Est./1 -> Switch/2
  Frame Status Conversion2/1 -> Out1/1

== system ofdm_13/OFDM Rx/BER Meas. ==
  In1 : Inport
  Bernoulli Random Binary Generator : commrandsrc2/Bernoulli Binary Generator  DialogController=commDDGCreate  DialogControllerArgs=DataTag1  SystemSampleTime=-1  P=0.5  seed=123  Ts=-1  frameBased=on  sampPerFrame=Bits_per_Frame  orient=off  outDataType=double
  Error Rate Calculation : commsink2/Error Rate Calculation  N=270  st_delay=810-180  cp_mode=Entire frame  subframe=[]  PMode=Port  WsName=ErrorVec  RsMode2=off  stop=off  numErr=100  maxBits=1e6
  Rectangular QAM Demodulator Baseband : commdigbbndam3/Rectangular QAM Demodulator Baseband  DialogController=commDDGCreate  DialogControllerArgs=DataTag2  M=4  PowType=Min. distance between symbols  MinDist=2  AvgPow=1  PeakPow=1  Ph=0  Dec=Binary  Mapping=[0:15]  OutType=Bit  DecType=Hard decision  VarSource=Dialog  Variance=1  outDtype1=Inherit via internal rule  outDtype2=Inherit via internal rule  derotateFactorWordLen=16  denormFactorWordLen=16  prodOutWordLen=32  prodOutRoundingMode=Floor  prodOutOverflowMode=Wrap  sumWordLen=32
  ber : Outport  OutDataType=sfix(16)  OutScaling=2^0  InitialOutput=nco_nominal
  wires:
  Rectangular QAM Demodulator Baseband/1 -> Error Rate Calculation/2
  Bernoulli Random Binary Generator/1 -> Error Rate Calculation/1
  In1/1 -> Rectangular QAM Demodulator Baseband/1
  Error Rate Calculation/1 -> ber/1

== system ofdm_13/OFDM Rx/Carrier Recovery  PI Controller ==
  Fine Correction : Inport
  Enable : EnablePort
  Add1 : Sum  OutDataType=sfix(16)  OutScaling=2^-10
  Add2 : Sum  OutDataType=sfix(16)  OutScaling=2^-10
  Delay1 : dspsigops/Delay  dly_unit=Samples  delay=1  ic_detail=off  dif_ic_for_ch=off  dif_ic_for_dly=off  ic=0  reset_popup=None
  P Gain : Gain  Gain=3  ParameterDataType=sfix(16)  ParameterScaling=2^0  OutDataType=sfix(16)  OutScaling=2^0
  PI Gain : Gain  Gain=-200  ParameterDataType=sfix(16)  ParameterScaling=2^0  OutDataType=sfix(16)  OutScaling=2^0
  Saturation : Saturate  UpperLimit=2000  LowerLimit=-2000  OutDataType=sfix(16)  OutScaling=2^0
  Saturation1 : Saturate  UpperLimit=2000  LowerLimit=-2000  OutDataType=sfix(16)  OutScaling=2^0
  Out : Outport
  wires:
  P Gain/1 -> Add2/1
  Add2/1 -> Saturation1/1
  Fine Correction/1 -> PI Gain/1
  PI Gain/1 -> P Gain/1, Add1/1
  Saturation/1 -> Add2/2, Delay1/1
  Add1/1 -> Saturation/1
  Delay1/1 -> Add1/2
  Saturation1/1 -> Out/1

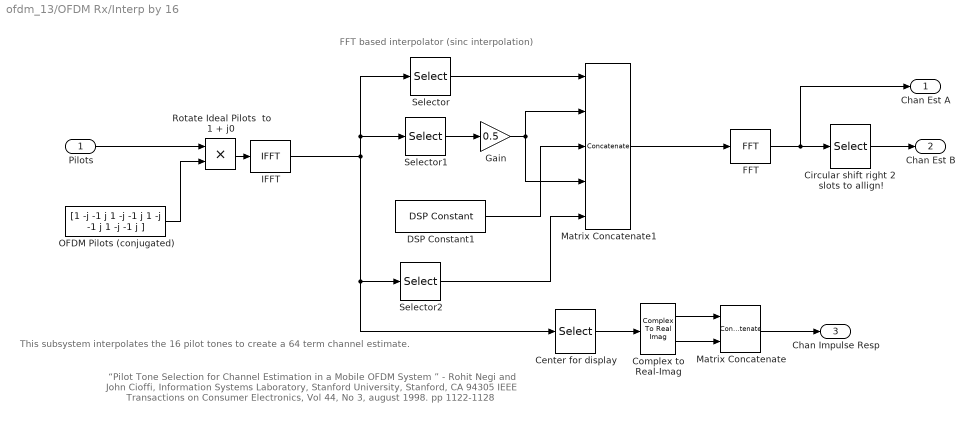
== system ofdm_13/OFDM Rx/Interp by 16 ==
  note: FFT based interpolator (sinc interpolation)
  note: This subsystem interpolates the 16 pilot
      |  tones to create a 64 term channel estimate.
  note: “Pilot Tone Selection for Channel Estimation in a Mobile OFDM System ”
      | -  Rohit Negi and John Cioffi, Information Systems Laboratory, Stanford University, Stanford, CA 94305
      | IEEE Transactions on Consumer Electronics, Vol 44, No 3, august 1998. pp 1122-1128
  Pilots : Inport
  "Center for display " : Selector  InputPortWidth=16  IndexOptions=Index vector (dialog)  Indices=[9:16 1:8]  OutputSizes=1
  Circular shift right 2  slots to allign! : Selector  InputPortWidth=64  IndexOptions=Index vector (dialog)  Indices=[63 64 1:62]  OutputSizes=1
  Complex to Real-Imag : ComplexToRealImag
  DSP Constant1 : dspobslib/DSP Constant  SystemSampleTime=-1  Value=zeros(47,1)  SampleMode=Discrete  discreteOutput=Sample-based  continuousOutput=Sample-based  sampTime=-1  framePeriod=2  dataType=Inherit from 'Constant value'  isSigned=on  wordLen=16  udDataType=sfix(16)  fracBitsMode=Best precision  numFracBits=15  InterpretAs1D=-inf  Ts=-inf  FramebasedOutput=-inf
  FFT : dspxfrm3/FFT  DialogController=dspDDGCreate  DialogControllerArgs=DataTag6  CompMethod=Table lookup  TableOpt=HYBRID  TableOptActive=Speed  BitRevOrder=off  InheritFFTLength=on  FFTLength=64  SkipNorm=off  roundingMode=Floor  overflowMode=off
  Gain : Gain  Gain=0.5  ParameterDataType=sfix(16)  ParameterScaling=2^0  OutDataType=sfix(16)  OutScaling=2^0
  IFFT : dspxfrm3/IFFT  DialogController=dspDDGCreate  DialogControllerArgs=DataTag7  CompMethod=Table lookup  TableOpt=HYBRID  TableOptActive=Speed  BitRevOrder=off  cs_in=off  SkipNorm=on  InheritFFTLength=on  FFTLength=64  mode=Complex  outSamplingMode=Frame based  roundingMode=Floor  overflowMode=off
  Matrix Concatenate : Concatenate  Mode=Multidimensional array  ConcatenateDimension=2
  Matrix Concatenate1 : Concatenate  NumInputs=5  Mode=Multidimensional array
  OFDM Pilots (conjugated) : Constant  Value="[1 -j -1 j    1 -j -1 j    1 -j -1 j    1 -j -1 j    ]"  OutDataType=sfix(16)  OutScaling=2^0  FramePeriod=-1
  Rotate Ideal Pilots  to 1 + j0 : Product  Inputs=**  OutDataType=sfix(16)  OutScaling=2^0  RndMeth=Zero
  Selector : Selector  InputPortWidth=16  IndexOptions=Index vector (dialog)  Indices=[1:8]  OutputSizes=1
  Selector1 : Selector  InputPortWidth=16  IndexOptions=Index vector (dialog)  Indices=9  OutputSizes=1
  Selector2 : Selector  InputPortWidth=16  IndexOptions=Index vector (dialog)  Indices=10:16  OutputSizes=1
  Chan Est A : Outport
  Chan Est B : Outport  Port=2
  Chan Impulse Resp : Outport  Port=3
  wires:
  Matrix Concatenate1/1 -> FFT/1
  Selector/1 -> Matrix Concatenate1/1
  Selector1/1 -> Gain/1
  DSP Constant1/1 -> Matrix Concatenate1/3
  Gain/1 -> Matrix Concatenate1/2, Matrix Concatenate1/4
  Selector2/1 -> Matrix Concatenate1/5
  FFT/1 -> Chan Est A/1, Circular shift right 2  slots to allign!/1
  IFFT/1 -> Selector/1, Selector1/1, Selector2/1, "Center for display "/1
  Complex to Real-Imag/1 -> Matrix Concatenate/1
  Complex to Real-Imag/2 -> Matrix Concatenate/2
  "Center for display "/1 -> Complex to Real-Imag/1
  Matrix Concatenate/1 -> Chan Impulse Resp/1
  Circular shift right 2  slots to allign!/1 -> Chan Est B/1
  Rotate Ideal Pilots  to 1 + j0/1 -> IFFT/1
  Pilots/1 -> Rotate Ideal Pilots  to 1 + j0/1
  OFDM Pilots (conjugated)/1 -> Rotate Ideal Pilots  to 1 + j0/2

== system ofdm_13/OFDM Rx/OFDM Receiver ==
  Received signal : Inport  OutDataType=sfix(16)  OutScaling=2^0
  FFT : dspxfrm3/FFT  DialogController=dspDDGCreate  DialogControllerArgs=DataTag8  CompMethod=Table lookup  TableOpt=HYBRID  TableOptActive=Speed  BitRevOrder=off  InheritFFTLength=on  FFTLength=64  SkipNorm=off  roundingMode=Floor  overflowMode=off
  Gain1 : Gain  Gain=1/Pilot_Level  ParameterDataType=sfix(16)  ParameterScaling=2^0  OutDataType=sfix(16)  OutScaling=2^0
  Gain2 : Gain  Gain=1/QAM_Level  ParameterDataType=sfix(16)  ParameterScaling=2^0  OutDataType=sfix(16)  OutScaling=2^0  SaturateOnIntegerOverflow=on  OutDataTypeStr=Inherit: Same as input  ParamDataTypeStr=Inherit: Same as input
  Remove Cyclic Prefix : Selector  InputPortWidth=80  IndexOptions=Index vector (dialog)  Indices=[17:80]  OutputSizes=1
  Remove pilots : Subsystem
  reorder : Selector  InputPortWidth=64  IndexOptions=Index vector (dialog)  Indices=[33:64 1:32]  OutputSizes=1
  Data : Outport  OutDataType=sfix(16)  OutScaling=2^0
  PIlots : Outport  Port=2  OutDataType=sfix(16)  OutScaling=2^0
  wires:
  FFT/1 -> reorder/1
  Received signal/1 -> Remove Cyclic Prefix/1
  Remove Cyclic Prefix/1 -> FFT/1
  Remove pilots/2(Pilots) -> Gain1/1
  Remove pilots/1(Data) -> Gain2/1
  Gain2/1 -> Data/1
  reorder/1 -> Remove pilots/1("  ")
  Gain1/1 -> PIlots/1

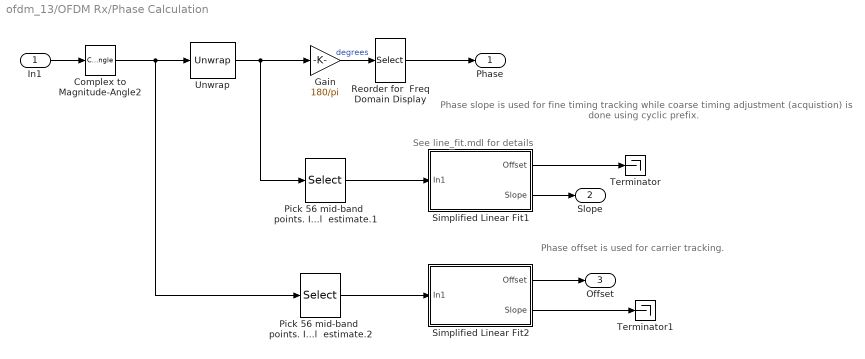
== system ofdm_13/OFDM Rx/Phase Calculation ==
  note: See line_fit.mdl for details
  note: Phase slope is used for fine
      | timing tracking while coarse timing adjustment
      | (acquistion) is done using cyclic prefix.
  note: Phase offset is used for carrier tracking.
  In1 : Inport
  Complex to Magnitude-Angle2 : ComplexToMagnitudeAngle  Output=Angle
  Gain : Gain  Gain=180/pi  ParameterDataType=sfix(16)  ParameterScaling=2^0  OutDataType=sfix(16)  OutScaling=2^0
  Pick 56 mid-band  points. Ignore end points of channel  estimate.1 : Selector  InputPortWidth=64  IndexOptions=Index vector (dialog)  Indices=[5:60]  OutputSizes=1
  Pick 56 mid-band  points. Ignore end points of channel  estimate.2 : Selector  InputPortWidth=64  IndexOptions=Index vector (dialog)  Indices=[5:60]  OutputSizes=1
  Reorder for  Freq Domain Display : Selector  InputPortWidth=64  IndexOptions=Index vector (dialog)  Indices=[33:64 1:32]  OutputSizes=1
  Simplified Linear Fit1 : Subsystem
  Simplified Linear Fit2 : Subsystem
  Terminator : Terminator
  Terminator1 : Terminator
  Unwrap : dspsigops/Unwrap  running=on  tol=pi*1.99 %1.9
  Phase : Outport
  Slope : Outport  Port=2
  Offset : Outport  Port=3
  wires:
  Complex to Magnitude-Angle2/1 -> Unwrap/1, Pick 56 mid-band  points. Ignore end points of channel  estimate.2/1
  In1/1 -> Complex to Magnitude-Angle2/1
  Gain/1 -> Reorder for  Freq Domain Display/1  "degrees"
  Reorder for  Freq Domain Display/1 -> Phase/1
  Pick 56 mid-band  points. Ignore end points of channel  estimate.1/1 -> Simplified Linear Fit1/1(In1)
  Simplified Linear Fit1/2(Slope) -> Slope/1
  Unwrap/1 -> Gain/1, Pick 56 mid-band  points. Ignore end points of channel  estimate.1/1
  Pick 56 mid-band  points. Ignore end points of channel  estimate.2/1 -> Simplified Linear Fit2/1(In1)
  Simplified Linear Fit2/1(Offset) -> Offset/1
  Simplified Linear Fit1/1(Offset) -> Terminator/1
  Simplified Linear Fit2/2(Slope) -> Terminator1/1

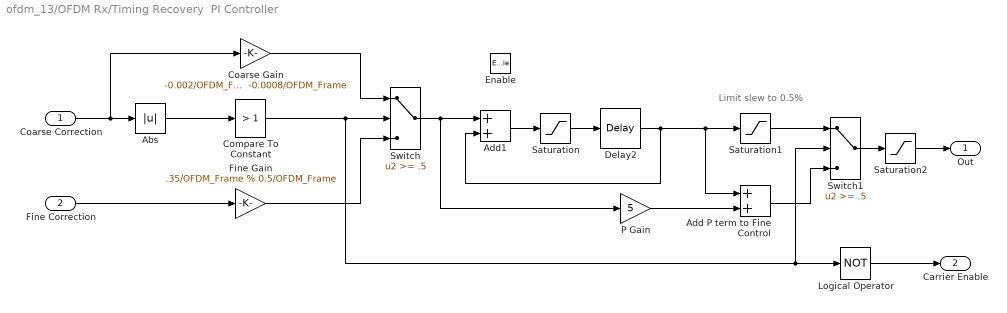
== system ofdm_13/OFDM Rx/Timing Recovery  PI Controller ==
  note: Limit slew to 0.5%
  Coarse Correction : Inport
  Fine Correction : Inport  Port=2
  Enable : EnablePort
  Abs : Abs  OutDataType=sfix(16)  OutScaling=2^0
  Add P term to Fine Control : Sum  OutDataType=sfix(16)  OutScaling=2^-10
  Add1 : Sum  OutDataType=sfix(16)  OutScaling=2^-10
  Coarse Gain : Gain  Gain="-0.002/OFDM_Frame   %  -0.0008/OFDM_Frame"  ParameterDataType=sfix(16)  ParameterScaling=2^0  OutDataType=sfix(16)  OutScaling=2^0
  Compare To Constant : simulink/Logic and Bit Operations/Compare To Constant  SystemSampleTime=-1  relop=>  const=1  LogicOutDataTypeMode=boolean  ZeroCross=off
  Delay2 : dspsigops/Delay  dly_unit=Samples  delay=1  ic_detail=off  dif_ic_for_ch=off  dif_ic_for_dly=off  ic=nco_nominal  reset_popup=None
  Fine Gain : Gain  Gain=.35/OFDM_Frame % 0.5/OFDM_Frame  ParameterDataType=sfix(16)  ParameterScaling=2^0  OutDataType=sfix(16)  OutScaling=2^0
  Logical Operator : Logic  Operator=NOT  AllPortsSameDT=off  OutDataTypeMode=boolean  OutDataTypeStr=boolean
  P Gain : Gain  Gain=5  ParameterDataType=sfix(16)  ParameterScaling=2^0  OutDataType=sfix(16)  OutScaling=2^0
  Saturation : Saturate  UpperLimit=nco_nominal*1.005  LowerLimit=nco_nominal*0.995  OutDataType=sfix(16)  OutScaling=2^0
  Saturation1 : Saturate  UpperLimit=nco_nominal*1.005  LowerLimit=nco_nominal*0.995  OutDataType=sfix(16)  OutScaling=2^0
  Saturation2 : Saturate  UpperLimit="nco_nominal*1.007  % 1.007"  LowerLimit="nco_nominal*0.993  % 0.993"  OutDataType=sfix(16)  OutScaling=2^0
  Switch : Switch  Threshold=.5  OutDataType=sfix(16)  OutScaling=2^0
  Switch1 : Switch  Threshold=.5  OutDataType=sfix(16)  OutScaling=2^0
  Out : Outport
  Carrier Enable : Outport  Port=2
  wires:
  Add1/1 -> Saturation/1
  Switch/1 -> Add1/1, P Gain/1
  Coarse Gain/1 -> Switch/1
  Fine Gain/1 -> Switch/3
  Coarse Correction/1 -> Abs/1, Coarse Gain/1
  Fine Correction/1 -> Fine Gain/1
  Abs/1 -> Compare To Constant/1
  Delay2/1 -> Add1/2, Add P term to Fine Control/1, Saturation1/1
  P Gain/1 -> Add P term to Fine Control/2
  Add P term to Fine Control/1 -> Switch1/3
  Switch1/1 -> Saturation2/1
  Compare To Constant/1 -> Switch/2, Switch1/2, Logical Operator/1
  Saturation2/1 -> Out/1
  Logical Operator/1 -> Carrier Enable/1
  Saturation/1 -> Delay2/1
  Saturation1/1 -> Switch1/1
